simulink model "Modelling_of_PMSM"  (R2021a)
settings: Solver=ode4  StartTime=0.0  StopTime=10/116  FixedStep=1e-7  RelTol=1e-3
InitFcn:
  | P=4;
  | Rs=2;
  | Ld=0.0125;
  | Lq=0.0057;
  | PhiPM=0.123;
undefined symbols (not defined in the file): DiscIntNeverNeededParam
libraries: autolibpmsminterior x1, spsabctodq0Lib x1, spsdq0toabcLib x1
settings Model: Creator=es-mostafamoh111  LastModifiedBy=Mostafa

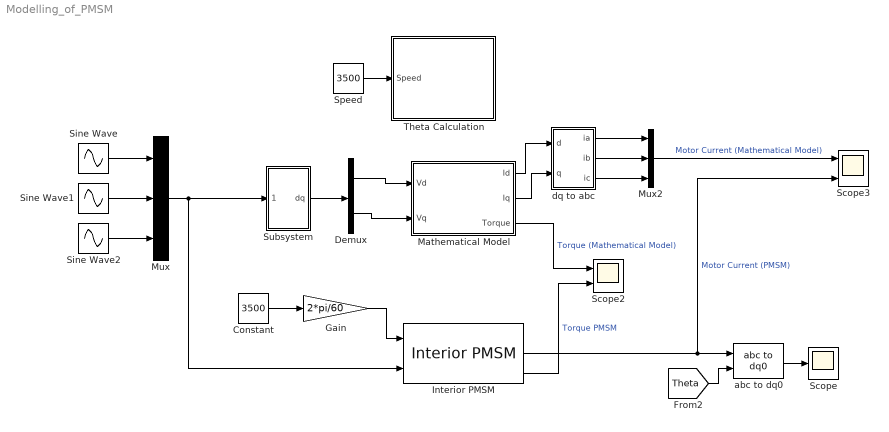
== system Modelling_of_PMSM ==
  Constant : Constant  Value=3500
  Demux : Demux  Outputs=2
  Gain : Gain  Gain=2*pi/60
  Interior PMSM : autolibpmsminterior/Interior PMSM  port_config=Speed  sim_type=Continuous  Ts=0.001  P=P/2  Rs=Rs  Ldq=[Ld Lq]  KConstText=Permanent flux linkage constant (lambda_pm):  lambda_pm=PhiPM  Ke=159.9771  mechanical=[0.002700,4.924e-4,0]  idq0=[0 0]  theta_init=0  omega_init=0  KConst=PhiPM  lambda_pm_calc=PhiPM  Kt=0.07  RefBlkName='autolibpmsminterior/Interior PMSM'  aMode=5
      settings: SourceProductBaseCode=PW,DR,MT,UV,VE
  Mathematical Model : Subsystem
  Mux : Mux  Inputs=3
  Mux2 : Mux  Inputs=3
  Scope : Scope
  Scope2 : Scope  NumInputPorts=2
  Scope3 : Scope  NumInputPorts=2
  Sine Wave : Sin  Amplitude=200*sqrt(2/3)  Frequency=733.0383  SampleTime=0
  Sine Wave1 : Sin  Amplitude=200*sqrt(2/3)  Frequency=733.0383  Phase=-2*pi/3  SampleTime=0
  Sine Wave2 : Sin  Amplitude=200*sqrt(2/3)  Frequency=733.0383  Phase=2*pi/3  SampleTime=0
  Speed : Constant  Value=3500
  Subsystem : Subsystem
  Theta Calculation : Subsystem
  abc to dq0 : spsabctodq0Lib/abc to dq0  Alignment=Aligned with phase A axis
  dq to abc : Subsystem
  wires:
  Sine Wave/1 -> Mux/1
  Sine Wave1/1 -> Mux/2
  Sine Wave2/1 -> Mux/3
  Constant/1 -> Gain/1
  Gain/1 -> Interior PMSM/1
  Demux/1 -> Mathematical Model/1(Vd)
  Mathematical Model/1(Id) -> dq to abc/1(d)
  Mathematical Model/2(Iq) -> dq to abc/2(q)
  Speed/1 -> Theta Calculation/1(Speed)
  Demux/2 -> Mathematical Model/2(Vq)
  Interior PMSM/2 -> abc to dq0/1, Scope3/2  "Motor Current (PMSM)"
  abc to dq0/1 -> Scope/1
  [Theta] -> abc to dq0/2
  Interior PMSM/3 -> Scope2/2  "Torque PMSM"
  Subsystem/1(dq) -> Demux/1
  Mux/1 -> Subsystem/1(abc), Interior PMSM/2
  dq to abc/2(ib) -> Mux2/2
  dq to abc/1(ia) -> Mux2/1
  dq to abc/3(ic) -> Mux2/3
  Mux2/1 -> Scope3/1  "Motor Current (Mathematical Model)"
  Mathematical Model/3(Torque) -> Scope2/1  "Torque (Mathematical Model)"

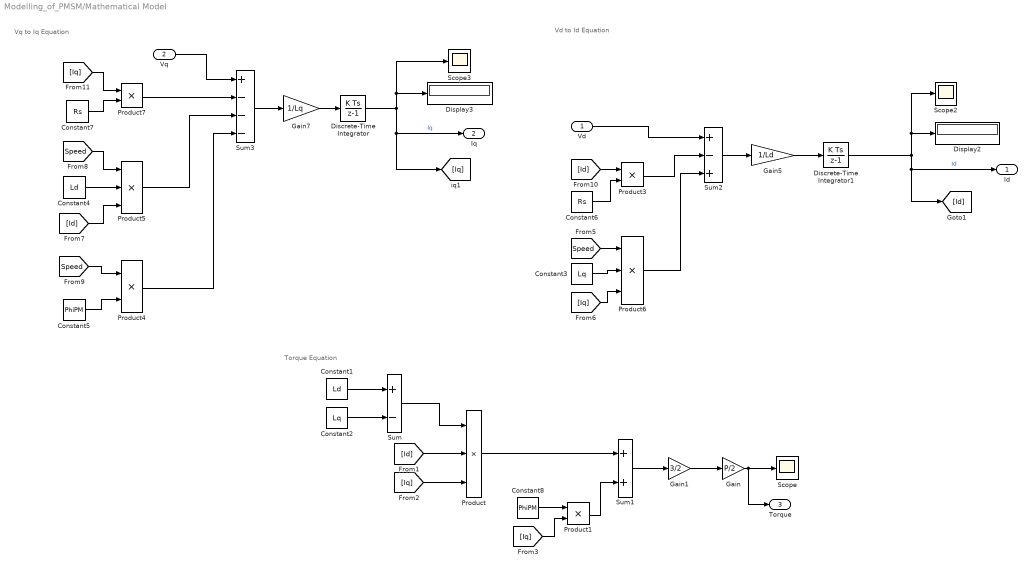
== system Modelling_of_PMSM/Mathematical Model ==
  note: Torque Equation
  note: Vq to Iq Equation
  note: Vd to Id Equation
  Vd : Inport
  Vq : Inport  Port=2
  Constant1 : Constant  Value=Ld
  Constant2 : Constant  Value=Lq
  Constant3 : Constant  Value=Lq
  Constant4 : Constant  Value=Ld
  Constant5 : Constant  Value=PhiPM
  Constant6 : Constant  Value=Rs
  Constant7 : Constant  Value=Rs
  Constant8 : Constant  Value=PhiPM
  Discrete-Time Integrator : DiscreteIntegrator  SampleTime=-1  ICPrevOutput=DiscIntNeverNeededParam  ICPrevScaledInput=DiscIntNeverNeededParam
  Discrete-Time Integrator1 : DiscreteIntegrator  SampleTime=-1  ICPrevOutput=DiscIntNeverNeededParam  ICPrevScaledInput=DiscIntNeverNeededParam
  Display2 : Display
  Display3 : Display
  Gain : Gain  Gain=P/2
  Gain1 : Gain  Gain=3/2
  Gain5 : Gain  Gain=1/Ld
  Gain7 : Gain  Gain=1/Lq
  Product : Product  Inputs=3
  Product{1,3..4,7} (4 alike) : Product
  Product5 : Product  Inputs=3
  Product6 : Product  Inputs=3
  Scope : Scope
  Scope2 : Scope
  Scope3 : Scope
  Sum : Sum  Inputs=+-
  Sum1 : Sum
  Sum2 : Sum  Inputs=+-+
  Sum3 : Sum  Inputs=+---
  Id : Outport
  Iq : Outport  Port=2
  Torque : Outport  Port=3
  wires:
  Discrete-Time Integrator1/1 -> [Id], Id/1, Scope2/1, Display2/1  "Id"
  Constant3/1 -> Product6/2
  [Speed] -> Product6/1
  Product3/1 -> Sum2/2
  Constant6/1 -> Product3/2
  Vd/1 -> Sum2/1
  Sum2/1 -> Gain5/1
  Gain5/1 -> Discrete-Time Integrator1/1
  [Id] -> Product3/1
  [Iq] -> Product6/3
  Product6/1 -> Sum2/3
  Discrete-Time Integrator/1 -> Iq/1, [Iq], Scope3/1, Display3/1  "Iq"
  Vq/1 -> Sum3/1
  [Speed] -> Product5/1
  Product7/1 -> Sum3/2
  Product4/1 -> Sum3/4
  [Iq] -> Product7/1
  Constant7/1 -> Product7/2
  [Speed] -> Product4/1
  Product5/1 -> Sum3/3
  Gain7/1 -> Discrete-Time Integrator/1
  Sum3/1 -> Gain7/1
  Constant4/1 -> Product5/2
  Constant5/1 -> Product4/2
  [Id] -> Product5/3
  Gain/1 -> Torque/1, Scope/1
  Gain1/1 -> Gain/1
  Sum1/1 -> Gain1/1
  Sum/1 -> Product/1
  Constant2/1 -> Sum/2
  Product/1 -> Sum1/1
  [Iq] -> Product1/2
  [Id] -> Product/2
  Product1/1 -> Sum1/2
  Constant1/1 -> Sum/1
  [Iq] -> Product/3
  Constant8/1 -> Product1/1

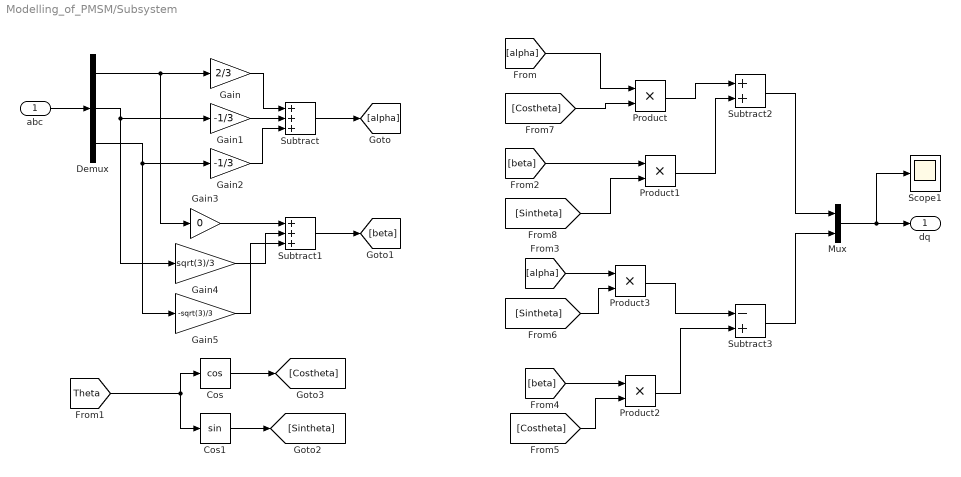
== system Modelling_of_PMSM/Subsystem ==
  abc : Inport
  Cos : Trigonometry  Operator=cos
  Cos1 : Trigonometry
  Demux : Demux  Outputs=3
  Gain : Gain  Gain=2/3
  Gain1 : Gain  Gain=-1/3
  Gain2 : Gain  Gain=-1/3
  Gain3 : Gain  Gain=0
  Gain4 : Gain  Gain=sqrt(3)/3
  Gain5 : Gain  Gain=-sqrt(3)/3
  Mux : Mux  Inputs=2
  Product{,1..3} (4 alike) : Product
  Scope1 : Scope
  Subtract : Sum  Inputs=+++
  Subtract1 : Sum  Inputs=+++
  Subtract2 : Sum
  Subtract3 : Sum  Inputs=-+
  dq : Outport
  wires:
  [Sintheta] -> Product1/2
  Cos1/1 -> [Sintheta]
  [Sintheta] -> Product3/2
  [Costheta] -> Product/2
  Subtract3/1 -> Mux/2
  Subtract2/1 -> Mux/1
  Product1/1 -> Subtract2/2
  [alpha] -> Product3/1
  Product3/1 -> Subtract3/1
  [beta] -> Product2/1
  Product2/1 -> Subtract3/2
  Cos/1 -> [Costheta]
  [beta] -> Product1/1
  Gain4/1 -> Subtract1/2
  Demux/3 -> Gain2/1, Gain5/1
  Gain5/1 -> Subtract1/3
  Gain2/1 -> Subtract/3
  [alpha] -> Product/1
  Demux/1 -> Gain3/1, Gain/1
  Gain/1 -> Subtract/1
  Subtract1/1 -> [beta]
  Product/1 -> Subtract2/1
  [Theta] -> Cos1/1, Cos/1
  [Costheta] -> Product2/2
  Gain1/1 -> Subtract/2
  abc/1 -> Demux/1
  Demux/2 -> Gain1/1, Gain4/1
  Gain3/1 -> Subtract1/1
  Subtract/1 -> [alpha]
  Mux/1 -> Scope1/1, dq/1

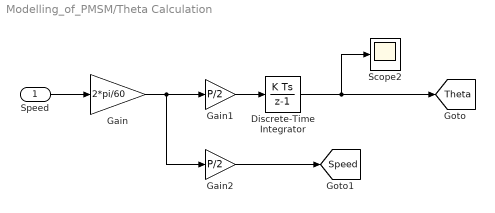
== system Modelling_of_PMSM/Theta Calculation ==
  Speed : Inport
  Discrete-Time Integrator : DiscreteIntegrator  SampleTime=-1  ICPrevOutput=DiscIntNeverNeededParam  ICPrevScaledInput=DiscIntNeverNeededParam
  Gain : Gain  Gain=2*pi/60
  Gain1 : Gain  Gain=P/2
  Gain2 : Gain  Gain=P/2
  Scope2 : Scope
  tag scope: Speed=global, Theta=global
  wires:
  Gain/1 -> Gain1/1, Gain2/1
  Speed/1 -> Gain/1
  Gain2/1 -> [Speed]
  Discrete-Time Integrator/1 -> [Theta], Scope2/1
  Gain1/1 -> Discrete-Time Integrator/1

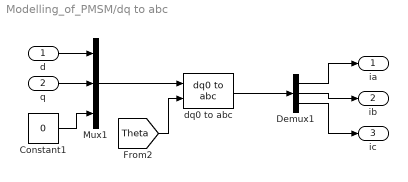
== system Modelling_of_PMSM/dq to abc ==
  d : Inport
  q : Inport  Port=2
  Constant1 : Constant  Value=0
  Demux1 : Demux  Outputs=3
  Mux1 : Mux  Inputs=3
  dq0 to abc : spsdq0toabcLib/dq0 to abc  Alignment=90 degrees behind phase A axis
  ia : Outport
  ib : Outport  Port=2
  ic : Outport  Port=3
  wires:
  dq0 to abc/1 -> Demux1/1
  Demux1/1 -> ia/1
  Mux1/1 -> dq0 to abc/1
  q/1 -> Mux1/2
  Demux1/2 -> ib/1
  d/1 -> Mux1/1
  Constant1/1 -> Mux1/3
  Demux1/3 -> ic/1
  [Theta] -> dq0 to abc/2
